simulink model "legacy_code_tool"  (R2019a)
settings: Solver=VariableStepAuto  StartTime=0.0  StopTime=10.0  RelTol=1e-3
undefined symbols (not defined in the file or in its folder): structParam
libraries: robotlib x2
settings Model: Creator=RUOBING  LastModifiedBy=RUOBING

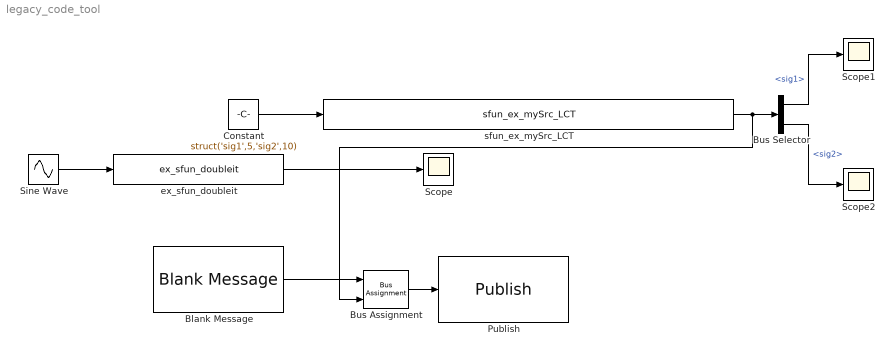
== system legacy_code_tool ==
  Blank Message : robotlib/Blank Message  messageClass=Message  entityType=std_msgs/UInt16  messageType=std_msgs/UInt16  SampleTime=inf
      settings: SourceProductBaseCode=RO
  Bus Assignment : BusAssignment  AssignedSignals=Data
  Bus Selector : BusSelector  OutputSignals=sig1,sig2
  Constant : Constant  Value=struct('sig1',5,'sig2',10)  OutDataTypeStr=Bus: sigStructType
  Publish : robotlib/Publish  topicSource=Specify your own  topic=/counter  messageType=std_msgs/UInt16  messageQueueLength=1
      settings: SourceProductBaseCode=RO
  Scope : Scope
  Scope1 : Scope
  Scope2 : Scope
  Sine Wave : Sin  SampleTime=0
  ex_sfun_doubleit : S-Function  FunctionName=ex_sfun_doubleit  SFunctionDeploymentMode=off  EnableBusSupport=off  mask(Legacy Function){SFunctionSpec=uint16 y1 = doubleIt(double u1), ShowSpec=on}
      mask prompts: ShowSpec "Display function specification"
      mask help:
      | This block allows you to call the legacy functions specified by the following Legacy Code Tool definition:
      | def.SFunctionName = 'ex_sfun_doubleit';
      | def.OutputFcnSpec = 'uint16 y1 = doubleIt(double u1)';
      | def.HeaderFiles = {'doubleIt.h'};
      mask Help: <p>This block was generated automatically by the Legacy Code Tool. For detailed help on this tool, call<a href="matlab:legacy_code('help')"> legacy_code('help')</a>.</p>
      mask Callback ShowSpec:
      | if strcmp(get_param(gcbh, 'ShowSpec'), 'on')
      |   set_param(gcbh, 'MaskDisplay', sprintf('fprintf(''%s'');', get_param(gcbh, 'SFunctionSpec')));
      | else
      |   set_param(gcbh, 'MaskDisplay', sprintf('fprintf(''%s'');', get_param(gcbh, 'FunctionName')));
      | end
      mask Display: fprintf('uint16 y1 = doubleIt(double u1)');
  sfun_ex_mySrc_LCT : S-Function  FunctionName=sfun_ex_mySrc_LCT  Parameters=SParameter1  SFunctionDeploymentMode=off  EnableBusSupport=off  mask(Legacy Function){SFunctionSpec=void myFcn(sigStructType u1[1], paramStructType p1[1], sigStructType y1[1]), SParameter1=structParam, ShowSpec=on}
      mask prompts: SParameter1 "P1:"; ShowSpec "Display function specification"
      mask help:
      | This block allows you to call the legacy functions specified by the following Legacy Code Tool definition:
      | def.SFunctionName = 'sfun_ex_mySrc_LCT';
      | def.OutputFcnSpec = 'void myFcn(sigStructType u1[1], paramStructType p1[1], sigStructType y1[1])';
      | def.HeaderFiles = {'ex_myTypes_LCT.h'};
      mask Help: <p>This block was generated automatically by the Legacy Code Tool. For detailed help on this tool, call<a href="matlab:legacy_code('help')"> legacy_code('help')</a>.</p>
      mask Callback ShowSpec:
      | if strcmp(get_param(gcbh, 'ShowSpec'), 'on')
      |   set_param(gcbh, 'MaskDisplay', sprintf('fprintf(''%s'');', get_param(gcbh, 'SFunctionSpec')));
      | else
      |   set_param(gcbh, 'MaskDisplay', sprintf('fprintf(''%s'');', get_param(gcbh, 'FunctionName')));
      | end
      mask Display: fprintf('void myFcn(sigStructType u1[1], paramStructType p1[1], sigStructType y1[1])');
  wires:
  Bus Assignment/1 -> Publish/1
  Blank Message/1 -> Bus Assignment/1
  ex_sfun_doubleit/1 -> Scope/1
  Sine Wave/1 -> ex_sfun_doubleit/1
  Bus Selector/2 -> Scope2/1  "<sig2>"
  sfun_ex_mySrc_LCT/1 -> Bus Assignment/2, Bus Selector/1
  Constant/1 -> sfun_ex_mySrc_LCT/1
  Bus Selector/1 -> Scope1/1  "<sig1>"
